simulink model "vrtut3"  (Simulink 6.0)
settings: Solver=ode45  StartTime=0.0  StopTime=Inf  RelTol=1e-3
libraries: vrlib x2
Description:
  | Tutorial model to be used for V-Realm authoring example in the User's manual.
  | After creating the virtual world according to the instructions in the manual, include the VR block
  | in the model and connect B1, B2 coordinates and S scaling to corresponding nodes in
  | the virtual world.
settings Model: CovMetricSettings=d  Creator=Danek  LastModifiedBy=Houska  ExtModeTrigMode=oneshot  ExtModeArmWhenConnect=off
settings DataIOCC: SaveOutput=off  SaveTime=off  SignalLoggingName=logsOut
settings OptimizationCC: BooleanDataType=off
settings DebuggingCC: CheckExecutionContextPreStartOutputMsg=on  CheckExecutionContextRuntimeOutputMsg=on  SolverPrmCheckMsg=none
settings HardwareCC: TargetUnknown=on
settings ModelReferenceCC: UpdateModelReferenceTargets=IfOutOfDate
settings GRTTargetCC: LifeSpan=inf
settings SFSimCC: SFSimApplyToAllLibs=on  SFSimBuildMode=Incremental

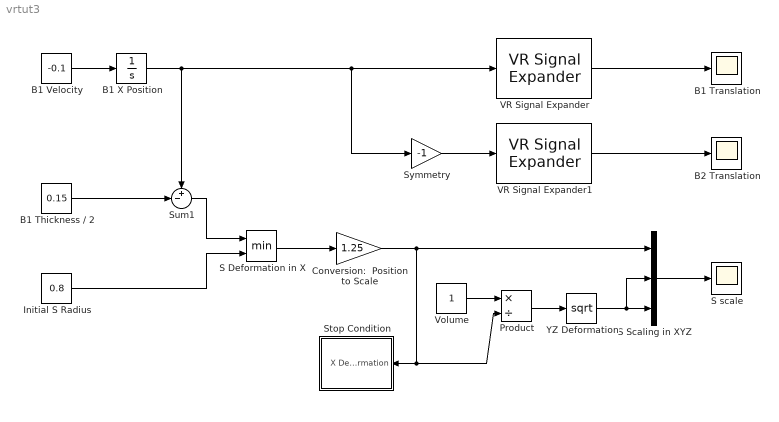
== system vrtut3 ==
  B1 Thickness / 2 : Constant  Value=0.15
  B1 Translation : Scope
  B1 Velocity : Constant  Value=-0.1
  B1 X Position : Integrator  InitialCondition=3  UpperSaturationLimit=Inf  LowerSaturationLimit=-Inf
  B2 Translation : Scope
  Conversion:  Position to Scale : Gain  Gain=1.25  SaturateOnIntegerOverflow=on
  Initial S Radius : Constant  Value=0.8
  Product : Product  Inputs=*/  SaturateOnIntegerOverflow=on  RndMeth=Zero  InputSameDT=on
  "S Deformation in X " : MinMax  Inputs=2  SaturateOnIntegerOverflow=on  InputSameDT=on
  S Scaling in XYZ : Mux  Inputs=3
  S scale : Scope
  Stop Condition : Subsystem  Orientation=left  EnableExecutionContextPropagation=on
  Sum1 : Sum  Inputs=+-|  SaturateOnIntegerOverflow=on  InputSameDT=on
  Symmetry : Gain  Gain=-1  SaturateOnIntegerOverflow=on
  VR Signal Expander : vrlib/VR Signal Expander  outwidth=3  outidx=1
  VR Signal Expander1 : vrlib/VR Signal Expander  outwidth=3  outidx=1
  Volume : Constant
  YZ Deformation : Math  Operator=sqrt  SaturateOnIntegerOverflow=on
  wires:
  Symmetry/1 -> VR Signal Expander1/1
  B1 X Position/1 -> Symmetry/1, VR Signal Expander/1, Sum1/1
  "S Deformation in X "/1 -> Conversion:  Position to Scale/1
  B1 Velocity/1 -> B1 X Position/1
  B1 Thickness / 2/1 -> Sum1/2
  Initial S Radius/1 -> "S Deformation in X "/2
  Sum1/1 -> "S Deformation in X "/1
  Conversion:  Position to Scale/1 -> Product/2, Stop Condition/1(X Deformation), S Scaling in XYZ/1
  Volume/1 -> Product/1
  Product/1 -> YZ Deformation/1
  YZ Deformation/1 -> S Scaling in XYZ/2, S Scaling in XYZ/3
  S Scaling in XYZ/1 -> S scale/1
  VR Signal Expander/1 -> B1 Translation/1
  VR Signal Expander1/1 -> B2 Translation/1

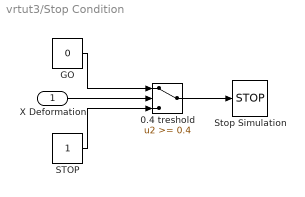
== system vrtut3/Stop Condition ==
  X Deformation : Inport  LatchInput=off
  0.4 treshold : Switch  Threshold=0.4  SaturateOnIntegerOverflow=on  InputSameDT=on
  GO : Constant  Value=0
  STOP : Constant
  Stop Simulation : Stop
  wires:
  X Deformation/1 -> 0.4 treshold/2
  GO/1 -> 0.4 treshold/1
  STOP/1 -> 0.4 treshold/3
  0.4 treshold/1 -> Stop Simulation/1
